simulink model "PID_controller_long_stage1_plot"  (R2019a)
settings: Solver=VariableStepAuto  StartTime=0.0  StopTime=80  FixedStep=1e-3  RelTol=1e-3
undefined symbols (not defined in the file): sys
libraries: aerolibactuator x1
settings Model: Creator=tyson  LastModifiedBy=tyson
settings DebuggingCC: InheritedTsInSrcMsg=none

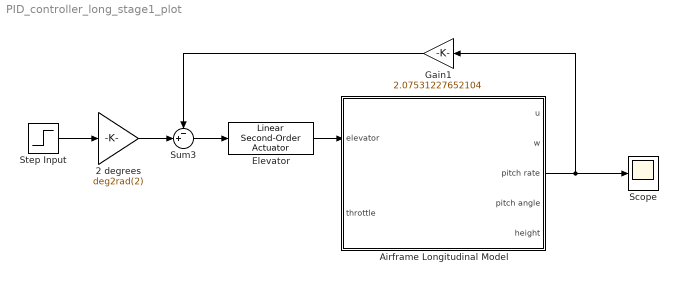
== system PID_controller_long_stage1_plot ==
  2 degrees : Gain  Gain=deg2rad(2)
  Airframe Longitudinal Model : Subsystem
      mask Display: image('/home/tyson/Dropbox/Academic/4th Year/ELEN4011/matlab/icons/airframe_long.png');
  Elevator : aerolibactuator/Linear Second-Order Actuator  wn_fin=actuators.naturalFreq  z_fin=actuators.dampingRatio  fin_act_0=0  fin_act_vel=0
      settings: SourceProductName=Aerospace Blockset  SourceProductBaseCode=AE
  Gain1 : Gain  Gain=2.07531227652104
  Scope : Scope
  Step Input : Step
  Sum3 : Sum  Inputs=-+|
  wires:
  Elevator/1 -> Airframe Longitudinal Model/1(elevator)
  Airframe Longitudinal Model/3(pitch rate) -> Gain1/1, Scope/1
  Sum3/1 -> Elevator/1
  Step Input/1 -> 2 degrees/1
  Gain1/1 -> Sum3/1
  2 degrees/1 -> Sum3/2

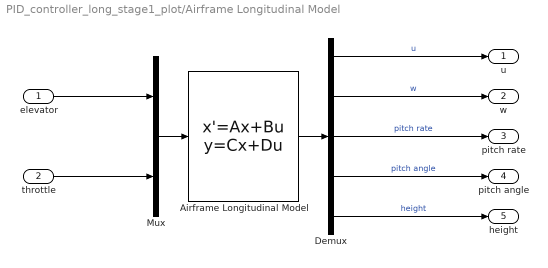
== system PID_controller_long_stage1_plot/Airframe Longitudinal Model ==
  elevator : Inport
  throttle : Inport  Port=2
  Airframe Longitudinal Model : StateSpace  A=sys.long.A  B=sys.long.B  C=sys.long.C  D=sys.long.D  InitialCondition=0
  Demux : Demux  Outputs=5
  Mux : Mux  Inputs=2
  u : Outport
  w : Outport  Port=2
  pitch rate : Outport  Port=3
  pitch angle : Outport  Port=4
  height : Outport  Port=5
  wires:
  throttle/1 -> Mux/2
  Demux/4 -> pitch angle/1  "pitch angle"
  Demux/3 -> pitch rate/1  "pitch rate"
  Mux/1 -> Airframe Longitudinal Model/1
  Airframe Longitudinal Model/1 -> Demux/1
  Demux/1 -> u/1  "u"
  Demux/2 -> w/1  "w"
  Demux/5 -> height/1  "height"
  elevator/1 -> Mux/1
